simulink model "ACS_2"  (Simulink 7.2)
settings: Solver=ode45  StartTime=0.0  StopTime=0.1  RelTol=1e-3
settings Model: Creator=Vano  LastModifiedBy=student
settings DebuggingCC: StrictBusMsg=ErrorLevel1

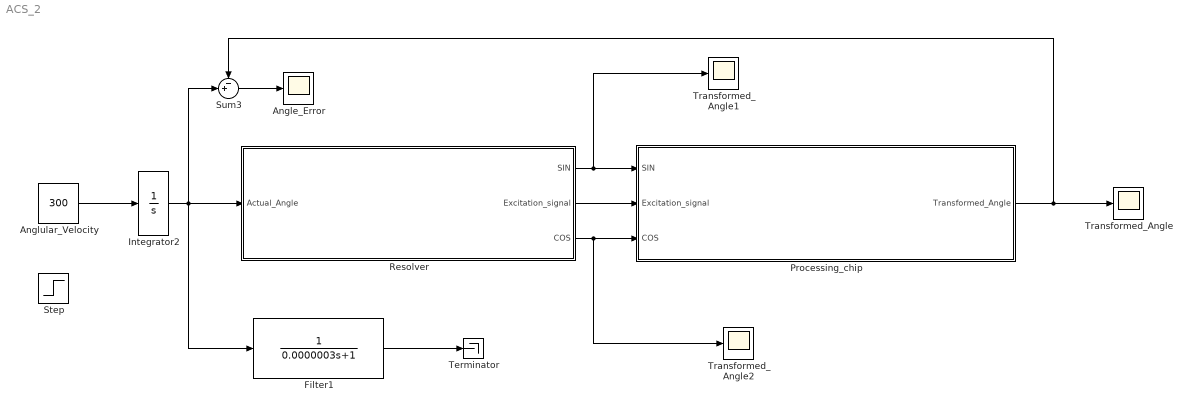
== system ACS_2 ==
  Angle_Error : Scope
      settings: TimeRange=0.1  YMin=0  YMax=0.35  SaveName=ScopeData10
  Anglular_Velocity : Constant  Value=300
  Filter1 : TransferFcn  Denominator=[0.0000003 1]
  Integrator2 : Integrator
  Processing_chip : Subsystem
  Resolver : Subsystem
  Step : Step  Time=0.5  SampleTime=0
  Sum3 : Sum  Inputs=-+|
  Terminator : Terminator
  Transformed_Angle : Scope
  Transformed_Angle1 : Scope
      settings: SaveName=ScopeData9
  Transformed_Angle2 : Scope
      settings: SaveName=ScopeData11
  wires:
  Sum3/1 -> Angle_Error/1
  Filter1/1 -> Terminator/1
  Processing_chip/1(Transformed_Angle) -> Transformed_Angle/1, Sum3/1
  Resolver/1(SIN) -> Processing_chip/1(SIN), Transformed_Angle1/1
  Resolver/3(COS) -> Processing_chip/3(COS), Transformed_Angle2/1
  Resolver/2(Excitation_signal) -> Processing_chip/2(Excitation_signal)
  Integrator2/1 -> Sum3/2, Resolver/1(Actual_Angle), Filter1/1
  Anglular_Velocity/1 -> Integrator2/1

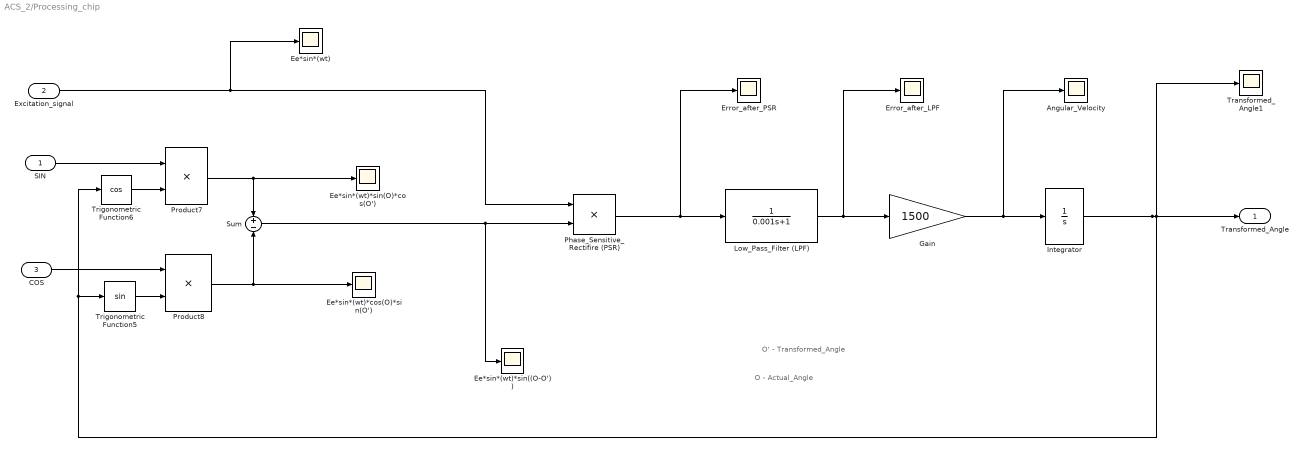
== system ACS_2/Processing_chip ==
  note: O' - Transformed_Angle
  note: O - Actual_Angle
  SIN : Inport
  Excitation_signal : Inport  Port=2
  COS : Inport  Port=3
  Angular_Velocity : Scope
      settings: TimeRange=0.006  YMin=0  YMax=350  SaveName=ScopeData2
  Ee*sin*(wt) : Scope
      settings: SaveName=ScopeData5
  Ee*sin*(wt)*cos(O)*sin(O') : Scope
      settings: SaveName=ScopeData7
  Ee*sin*(wt)*sin((O-O')) : Scope
      settings: SaveName=ScopeData4
  Ee*sin*(wt)*sin(O)*cos(O') : Scope
      settings: SaveName=ScopeData6
  Error_after_LPF : Scope
      settings: TimeRange=0.006  YMin=0  YMax=350  SaveName=ScopeData8
  Error_after_PSR : Scope
      settings: TimeRange=0.5  YMin=-1  YMax=1  SaveName=ScopeData3
  Gain : Gain  Gain=1500
  Integrator : Integrator
  Low_Pass_Filter (LPF) : TransferFcn  Denominator=[0.001 1]
  Phase_Sensitive_Rectifire (PSR) : Product  RndMeth=Zero
  Product7 : Product  RndMeth=Zero
  Product8 : Product  RndMeth=Zero
  Sum : Sum  Inputs=+-
  Transformed_Angle1 : Scope
      settings: YMin=0.19875  YMax=0.20125
  Trigonometric Function5 : Trigonometry
  Trigonometric Function6 : Trigonometry  Operator=cos
  Transformed_Angle : Outport
  wires:
  Trigonometric Function6/1 -> Product7/2
  Trigonometric Function5/1 -> Product8/2
  Product7/1 -> Sum/1, Ee*sin*(wt)*sin(O)*cos(O')/1
  Product8/1 -> Sum/2, Ee*sin*(wt)*cos(O)*sin(O')/1
  SIN/1 -> Product7/1
  COS/1 -> Product8/1
  Excitation_signal/1 -> Phase_Sensitive_Rectifire (PSR)/1, Ee*sin*(wt)/1
  Phase_Sensitive_Rectifire (PSR)/1 -> Low_Pass_Filter (LPF)/1, Error_after_PSR/1
  Sum/1 -> Phase_Sensitive_Rectifire (PSR)/2, Ee*sin*(wt)*sin((O-O'))/1
  Low_Pass_Filter (LPF)/1 -> Gain/1, Error_after_LPF/1
  Gain/1 -> Integrator/1, Angular_Velocity/1
  Integrator/1 -> Trigonometric Function6/1, Trigonometric Function5/1, Transformed_Angle1/1, Transformed_Angle/1

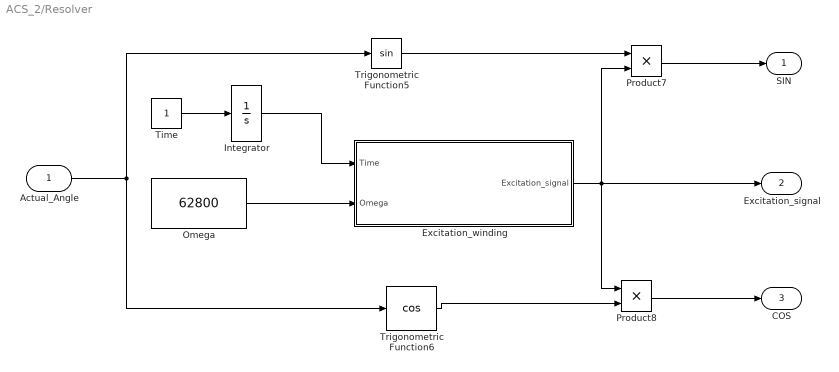
== system ACS_2/Resolver ==
  Actual_Angle : Inport
  Excitation_winding : Subsystem
  Integrator : Integrator
  Omega : Constant  Value=62800
  Product7 : Product  RndMeth=Zero
  Product8 : Product  RndMeth=Zero
  Time : Constant
  Trigonometric Function5 : Trigonometry
  Trigonometric Function6 : Trigonometry  Operator=cos
  SIN : Outport
  Excitation_signal : Outport  Port=2
  COS : Outport  Port=3
  wires:
  Time/1 -> Integrator/1
  Integrator/1 -> Excitation_winding/1(Time)
  Omega/1 -> Excitation_winding/2(Omega)
  Actual_Angle/1 -> Trigonometric Function6/1, Trigonometric Function5/1
  Trigonometric Function6/1 -> Product8/2
  Trigonometric Function5/1 -> Product7/1
  Excitation_winding/1(Excitation_signal) -> Product7/2, Product8/1, Excitation_signal/1
  Product7/1 -> SIN/1
  Product8/1 -> COS/1

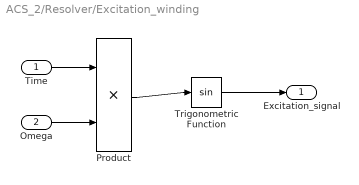
== system ACS_2/Resolver/Excitation_winding ==
  Time : Inport
  Omega : Inport  Port=2
  Product : Product  RndMeth=Zero
  Trigonometric Function : Trigonometry
  Excitation_signal : Outport
  wires:
  Omega/1 -> Product/2
  Trigonometric Function/1 -> Excitation_signal/1
  Time/1 -> Product/1
  Product/1 -> Trigonometric Function/1
